simulink model "Safety_filter_taskspace_run_FxTISMC"  (R2022a)
settings: Solver=ode4  StartTime=0.0  StopTime=30  FixedStep=0.01  RelTol=1e-3
libraries: simulink x1
settings Model: PacingRate=0.500000  Creator=14244039  LastModifiedBy=40335991
settings DebuggingCC: UnconnectedInputMsg=warning  UnconnectedOutputMsg=warning  UnconnectedLineMsg=warning  UnderSpecifiedDimensionMsg=warning
settings RTWCC: DLArmComputeVersion=19.05

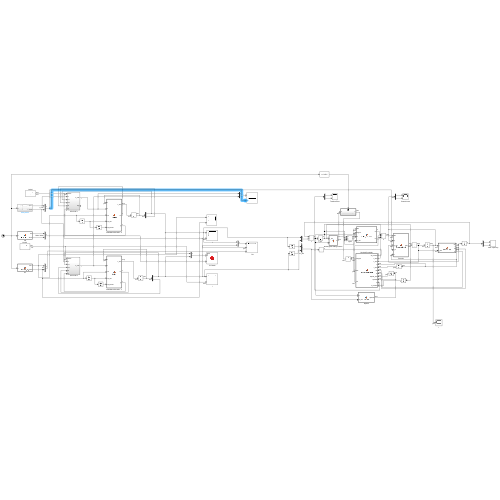
[thumbnail: Simulink's stored preview of the top-level diagram]
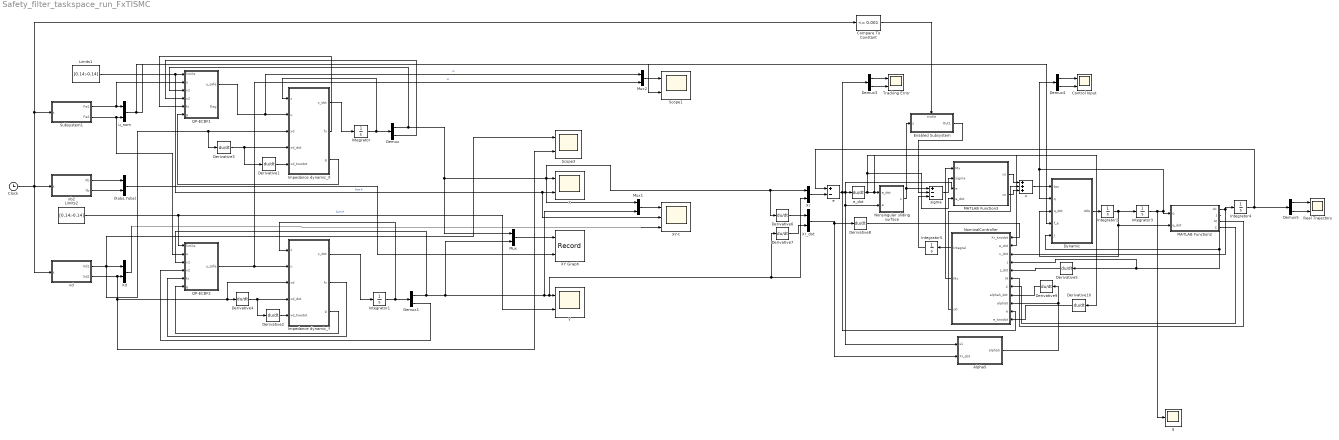
== system Safety_filter_taskspace_run_FxTISMC ==
  " Tracking Error" : Scope  NumInputPorts=2
  (Xobs,Yobs) : Mux  Inputs=2
  AlphaS : MATLAB Function  TreatAsAtomicUnit=on
  Clock : Clock
  Compare To Constant : simulink/Logic and Bit Operations/Compare To Constant  relop=<=  const=0.001  OutDataTypeStr=boolean
  Control Input : Scope  NumInputPorts=2
  Demux{,1,3..5} (5 alike) : Demux  Outputs=2
  Derivative{1..10} (10 alike) : Derivative
  Dynamic : MATLAB Function  TreatAsAtomicUnit=on
  Enabled Subsystem : Subsystem  TreatAsAtomicUnit=on
  Impedance dynamic_X : MATLAB Function  TreatAsAtomicUnit=on
  Impedance dynamic_Y : MATLAB Function  TreatAsAtomicUnit=on
  Integrator : Integrator  InitialCondition=[0.109;0]
  Integrator1 : Integrator  InitialCondition=[0;0]
  Integrator2 : Integrator
  Integrator3 : Integrator  InitialCondition=[0.5236;2.0944]
  Integrator4 : Integrator  InitialCondition=[0.14;0]
  Integrator5 : Integrator  InitialCondition=[0.0001;0.0001]
  Limits1 : Constant  Value=[0.14;-0.14]  VectorParams1D=off  SampleTime=-1
  Limits2 : Constant  Value=[0.14;-0.14]  VectorParams1D=off  SampleTime=-1
  MATLAB Function2 : MATLAB Function  TreatAsAtomicUnit=on
  MATLAB Function3 : MATLAB Function  TreatAsAtomicUnit=on
  Mux : Mux  Inputs=2
  Mux1 : Mux  Inputs=2
  Mux2 : Mux  Inputs=2
  NominalController : MATLAB Function  TreatAsAtomicUnit=on
  Nonsingular sliding surface : MATLAB Function  TreatAsAtomicUnit=on
  QP-ECBF1 : Subsystem
  QP-ECBF2 : Subsystem
  Real Trajectory : Scope  NumInputPorts=2
  Scope1 : Scope  NumInputPorts=2
  Scope3 : Scope  NumInputPorts=2
  Subsystem1 : Subsystem
  X : Scope  NumInputPorts=2
  XY Graph : Record  VariableName=Traj  RecordToWorkspace=on  FileSettingsInternal="{\"entries\":[{\"content\":{\"excelSettings\":{\"content\":{},\"type\":\"Streamout.ExcelSettings\"}},\"type\":\"Streamout.FileSettingStorage\",\"uuid\":\"dea1f68e-51ea-4f94-ad75-dcaf29079ec1\"}],\"packageUris\":[\"http://schema.mathworks.com/mf0/streamout_blocks/R2020a\"],\"version\":\"1.0\"}"  Layout=[1 1]  SignalsInternal="{\"entries\":[{\"content\":{\"signals\":[{\"content\":{\"blockPath\":[\"Safety_filter_taskspace_run_FxTISMC/XY Graph\"],\"channel\":[],\"dimensions\":[2],\"domain\":\"Safety_filter_taskspace_run_FxTISMC/XY Graph\",\"hasChildren\":true,\"lineColor\":\"#0072bd\",\"plots\":[],\"port\":1,\"sid\":[\"\"],\"signalID\":23698,\"signalName\":\"Mux\"},\"type\":\"RecordBlkView.Signal\",\"uuid\":\"0a4beed2-2c3d-4c2f-aacd-e662c2a4948f\"},{\"content\":{\"blockPath\":[\"Safety_filter_taskspace_run_FxTISMC/XY Graph\"],\"channel\":[1],\"dimensions\":[2],\"domain\":\"Safety_filter_taskspace_run_FxTISMC/XY Graph\",\"lineColor\":\"#4dbeee\",\"parentID\":23698,\"plots\":[1],\"port\":1,\"sid\":[\"\"],\"signalID\":23699,\"signalName\":\"Mux\"},\"type\":\"RecordBlkView.Signal\",\"uuid\":\"3713fb18-b151-4fd8-8a41-96ba99eca4e4\"},{\"content\":{\"blockPath\":[\"Safety_filter_taskspace_run_FxTISMC/XY Graph\"],\"channel\":[],\"dimensions\":[2],\"domain\":\"Safety_filter_taskspace_run_FxTISMC/XY Graph\",\"hasChildren\":true,\"lineColor\":\"#edb120\",\"plots\":[],\"port\":2,\"sid\":[\"\"],\"signalID\":23703,\"signalName\":\"(Xobs,Yobs)\"},\"type\":\"RecordBlkView.Signal\",\"uuid\":\"6070feb2-4c26-4461-aa6d-6878fe9a321b\"},{\"content\":{\"blockPath\":[\"Safety_filter_taskspace_run_FxTISMC/XY Graph\"],\"channel\":[1],\"dimensions\":[2],\"domain\":\"Safety_filter_taskspace_run_FxTISMC/XY Graph\",\"lineColor\":\"#139fff\",\"parentID\":23703,\"plots\":[],\"port\":2,\"sid\":[\"\"],\"signalID\":23704,\"signalName\":\"(Xobs,Yobs)\"},\"type\":\"RecordBlkView.Signal\",\"uuid\":\"40400d7a-2fa8-4b38-a7ba-519d3c7263bf\"},{\"content\":{\"blockPath\":[\"Safety_filter_taskspace_run_FxTISMC/XY Graph\"],\"channel\":[2],\"dimensions\":[2],\"domain\":\"Safety_filter_taskspace_run_FxTISMC/XY Graph\",\"lineColor\":\"#ff6929\",\"parentID\":23698,\"plots\":[1],\"port\":1,\"sid\":[\"\"],\"signalID\":23709,\"signalName\":\"Mux\"},\"type\":\"RecordBlkView.Signal\",\"uuid\":\"780f58a9-210e-4d63-889b-484a7d57ccdb\"},{\"content\":{\"blockPath\":[\"Safety_filter_taskspace_run_FxTISMC/XY Graph\"],\"channel\":[2],\"dimensions\":[2],\"domain\":\"Safety_filter_taskspace_run_FxTISMC/XY Graph\",\"lineColor\":\"#b746ff\",\"parentID\":23703,\"plots\":[],\"port\":2,\"sid\":[\"\"],\"signalID\":23710,\"signalName\":\"(Xobs,Yobs)\"},\"type\":\"RecordBlkView.Signal\",\"uuid\":\"fbf2c2ca-e6c1-4b56-8b91-8f9b3b0d1395\"}]},\"type\":\"RecordBlkView.InputSignals\",\"uuid\":\"3059aa5f-a949-4de9-9f01-a09f95338b02\"}],\"packageUris\":[\"http://schema.mathworks.com/mf0/streamout_blocks/R2020a\"],\"version\":\"1.0\"}"  VisualizationBindings="{\"xyplotplugin\":{\"info\":[{\"series\":[{\"bindingParametersList\":[{\"parameter\":\"X-Axis\",\"signalID\":23699,\"signalName\":\"Mux(1)\"},{\"parameter\":\"Y-Axis\",\"signalID\":23709,\"signalName\":\"Mux(2)\"}],\"seriesID\":34366}],\"subplotID\":1}]}}"  CompatibilityTag=XY  st=-1
  XY-t : Scope  NumInputPorts=3
  Xd : Mux  Inputs=2
  Xr : Mux  Inputs=2
  Xr_dot : Mux  Inputs=2
  Y : Scope  NumInputPorts=2
  e : Sum  Inputs=+-
  e_dot : Derivative
  q : Scope
  sigma : Sum  Inputs=+--
  u : Sum  Inputs=+++
  u_nom : Mux  Inputs=2
  xb2 : MATLAB Function  TreatAsAtomicUnit=on
  xd : MATLAB Function  TreatAsAtomicUnit=on
  wires:
  xd/1(Xd1) -> Scope3/1, Impedance dynamic_X/3(xd), Derivative3/1, Xd/1
  Subsystem1/1(Fe1) -> QP-ECBF1/2(u), u_nom/1
  Clock/1 -> xd/1(t), xb2/1(t), Compare To Constant/1, Subsystem1/1(t)
  Derivative3/1 -> Impedance dynamic_X/4(xd_dot), Derivative1/1
  Derivative1/1 -> Impedance dynamic_X/5(xd_twodot)
  Impedance dynamic_X/1(x_dot) -> Integrator/1
  Integrator/1 -> Demux/1, Impedance dynamic_X/1(x)
  Demux/1 -> QP-ECBF1/3(x1), Mux/1, Mux1/1, X/1, Derivative6/1, Xr/1
  Limits1/1 -> XY-t/2, X/2, QP-ECBF1/1(limits)  "lim+"
  Demux/2 -> QP-ECBF1/4(x2)
  QP-ECBF1/1(u_safe) -> Mux2/1, Impedance dynamic_X/2(u)  "u"
  Impedance dynamic_X/2(fx) -> QP-ECBF1/5(fx)
  Impedance dynamic_X/3(g) -> QP-ECBF1/6(g)
  Impedance dynamic_Y/3(g) -> QP-ECBF2/6(g)
  Impedance dynamic_Y/2(fx) -> QP-ECBF2/5(fx)
  QP-ECBF2/1(u_safe) -> Mux2/2, Impedance dynamic_Y/2(u)  "u"
  Demux1/2 -> QP-ECBF2/4(x2)
  Demux1/1 -> QP-ECBF2/3(x1), Mux1/2, Derivative7/1, Xr/2, Y/1, Mux/2
  xd/2(Xd2) -> Scope3/2, Impedance dynamic_Y/3(xd), Derivative4/1, Xd/2
  Limits2/1 -> Y/2, QP-ECBF2/1(limits)  "lim+"
  Impedance dynamic_Y/1(x_dot) -> Integrator1/1
  Derivative4/1 -> Impedance dynamic_Y/4(xd_dot), Derivative2/1
  Derivative2/1 -> Impedance dynamic_Y/5(xd_twodot)
  Integrator1/1 -> Demux1/1, Impedance dynamic_Y/1(x)
  Subsystem1/2(Fe2) -> QP-ECBF2/2(u), u_nom/2
  xb2/1(Xb) -> (Xobs,Yobs)/1
  xb2/2(Yb) -> (Xobs,Yobs)/2
  Mux/1 -> XY Graph/1
  (Xobs,Yobs)/1 -> XY Graph/2
  Mux1/1 -> XY-t/1
  Xd/1 -> XY-t/3
  Mux2/1 -> Scope1/1
  u_nom/1 -> Dynamic/4(f_e), Scope1/2
  Xr/1 -> e/2
  Demux4/2 -> Control Input/2
  Nonsingular sliding surface/1(s) -> Enabled Subsystem/1(s), sigma/1
  Demux3/1 -> " Tracking Error"/1
  Integrator5/1 -> sigma/3
  NominalController/1(Integral) -> Integrator5/1
  Demux5/2 -> Real Trajectory/2
  Compare To Constant/1 -> Enabled Subsystem/Enable
  Demux3/2 -> " Tracking Error"/2
  Derivative7/1 -> Xr_dot/2
  e_dot/1 -> MATLAB Function3/4(e_dot), Derivative10/1, NominalController/2(e_dot), Nonsingular sliding surface/1(e_dot)
  MATLAB Function3/1(us) -> u/1
  Derivative5/1 -> NominalController/5(J_dot)
  Integrator2/1 -> MATLAB Function2/2(q_dot), Dynamic/3(q_dot), Integrator3/1
  Demux5/1 -> Real Trajectory/1
  MATLAB Function2/2(J) -> Dynamic/5(J), NominalController/4(J), Derivative5/1
  Integrator3/1 -> q/1, Demux4/1, Dynamic/2(q), MATLAB Function2/1(q)
  sigma/1 -> MATLAB Function3/2(sigma)
  Integrator4/1 -> Demux5/1, e/1
  Enabled Subsystem/1(Out1) -> sigma/2
  Derivative10/1 -> NominalController/11(e_twodot)
  MATLAB Function2/4(C) -> NominalController/7(C)
  NominalController/3(u0) -> u/2
  Xr_dot/1 -> AlphaS/2(Xr_dot), Derivative8/1
  Derivative9/1 -> NominalController/8(alphaS_dot)
  AlphaS/1(alphaS) -> Derivative9/1, NominalController/9(alphaS)
  MATLAB Function2/3(M) -> NominalController/6(M)
  MATLAB Function3/2(uc) -> u/3
  Derivative6/1 -> Xr_dot/1
  Dynamic/1(ddq) -> Integrator2/1
  NominalController/2(Mx) -> MATLAB Function3/1(Mx)
  Derivative8/1 -> NominalController/1(Xr_twodot)
  e/1 -> Demux3/1, e_dot/1, MATLAB Function3/3(e), AlphaS/1(s1), Nonsingular sliding surface/2(e), NominalController/10(e)
  MATLAB Function2/1(dx) -> Integrator4/1, NominalController/3(x_dot)
  u/1 -> Dynamic/1(tau)
  Demux4/1 -> Control Input/1

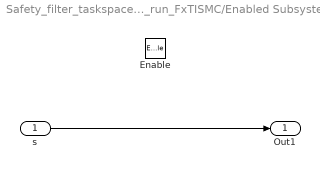
== system Safety_filter_taskspace_run_FxTISMC/Enabled Subsystem ==
  s : Inport
  Enable : EnablePort
  Out1 : Outport  InitialOutput=0  VectorParamsAs1DForOutWhenUnconnected=off
  wires:
  s/1 -> Out1/1

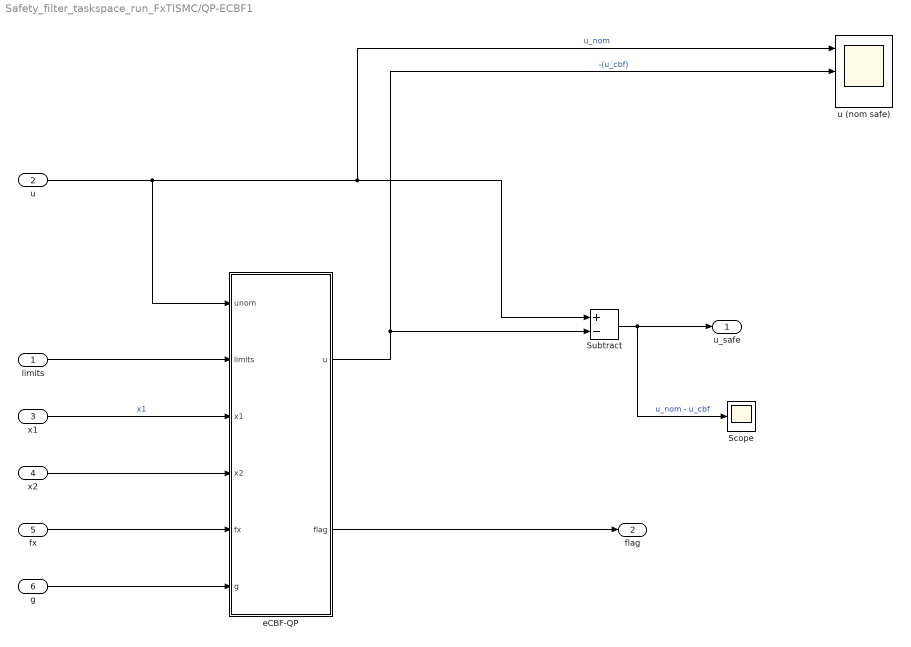
== system Safety_filter_taskspace_run_FxTISMC/QP-ECBF1 ==
  limits : Inport
  u : Inport  Port=2
  x1 : Inport  Port=3
  x2 : Inport  Port=4
  fx : Inport  Port=5
  g : Inport  Port=6
  Scope : Scope
  Subtract : Sum  Inputs=+-
  eCBF-QP : MATLAB Function  TreatAsAtomicUnit=on
  u (nom safe) : Scope  NumInputPorts=3
  u_safe : Outport
  flag : Outport  Port=2
  wires:
  x2/1 -> eCBF-QP/4(x2)
  limits/1 -> eCBF-QP/2(limits)
  u/1 -> eCBF-QP/1(unom), Subtract/1, u (nom safe)/1  "u_nom"
  x1/1 -> eCBF-QP/3(x1)  "x1"
  eCBF-QP/1(u) -> Subtract/2, u (nom safe)/2  "-(u_cbf)"
  Subtract/1 -> u_safe/1, Scope/1  "u_nom - u_cbf"
  fx/1 -> eCBF-QP/5(fx)
  g/1 -> eCBF-QP/6(g)
  eCBF-QP/2(flag) -> flag/1

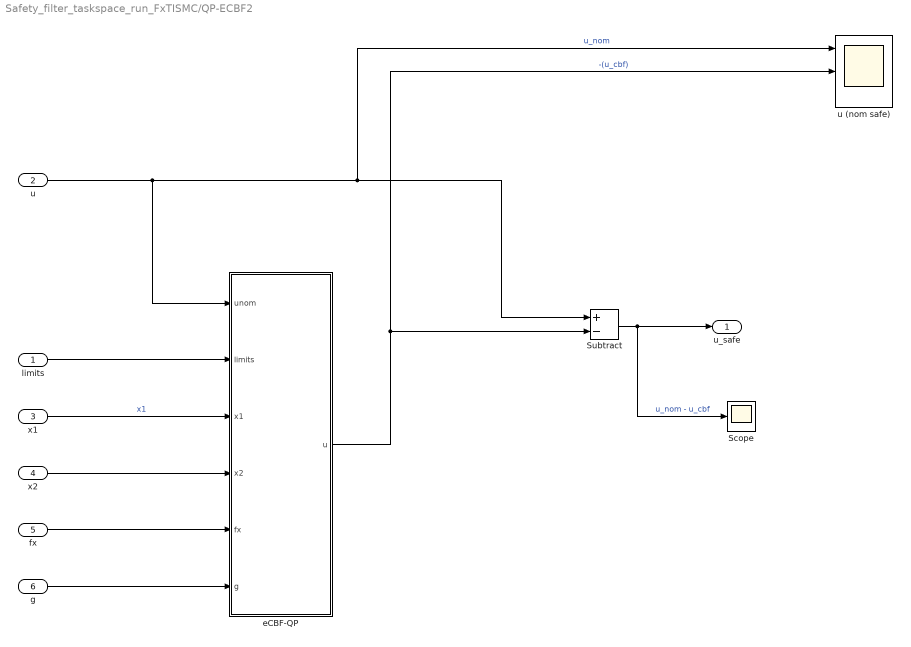
== system Safety_filter_taskspace_run_FxTISMC/QP-ECBF2 ==
  limits : Inport
  u : Inport  Port=2
  x1 : Inport  Port=3
  x2 : Inport  Port=4
  fx : Inport  Port=5
  g : Inport  Port=6
  Scope : Scope
  Subtract : Sum  Inputs=+-
  eCBF-QP : MATLAB Function  TreatAsAtomicUnit=on
  u (nom safe) : Scope  NumInputPorts=3
  u_safe : Outport
  wires:
  x2/1 -> eCBF-QP/4(x2)
  limits/1 -> eCBF-QP/2(limits)
  u/1 -> eCBF-QP/1(unom), Subtract/1, u (nom safe)/1  "u_nom"
  x1/1 -> eCBF-QP/3(x1)  "x1"
  eCBF-QP/1(u) -> Subtract/2, u (nom safe)/2  "-(u_cbf)"
  Subtract/1 -> u_safe/1, Scope/1  "u_nom - u_cbf"
  fx/1 -> eCBF-QP/5(fx)
  g/1 -> eCBF-QP/6(g)

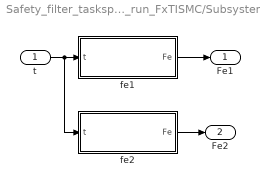
== system Safety_filter_taskspace_run_FxTISMC/Subsystem1 ==
  t : Inport
  fe1 : MATLAB Function  TreatAsAtomicUnit=on
  fe2 : MATLAB Function  TreatAsAtomicUnit=on
  Fe1 : Outport
  Fe2 : Outport  Port=2
  wires:
  fe1/1(Fe) -> Fe1/1
  fe2/1(Fe) -> Fe2/1
  t/1 -> fe2/1(t), fe1/1(t)

== matlab function Safety_filter_taskspace_run_FxTISMC/Dynamic ==
  data: tau input size=[2 1]; ddq output size=[2 1]; q input size=[2 1]; q_dot input size=[2 1]; f_e input; J input
function ddq  = TwoLinkRobot(tau,q,q_dot,f_e,J)
L = [0.3, 0.3];
m = [1.5, 1];
g = 9.8;

M = [m(2)*L(2)^2+2*m(2)*L(1)*L(2)*cos(q(2))+(m(1)+m(2))*L(1)^2, m(2)*L(2)^2+m(2)*L(1)*L(2)*cos(q(2));
    m(2)*L(2)^2+m(2)*L(1)*L(2)*cos(q(2)), m(2)*L(2)^2];
C = [-2*m(2)*L(1)*L(2)*sin(q(2))*q_dot(2), -m(2)*L(1)*L(2)*sin(q(2)); 
    m(2)*L(1)*L(2)*sin(q(2))*q_dot(1), 0];

F=[2*cos(q(1))*sin(q(2))+5*cos(q(1))^2;-2*cos(q(1))*sin(q(2))-5*cos(q(1))^2];

tau_e = (J')*f_e;
ddq = M\(-C*q_dot-F + tau + tau_e);

end

== matlab function Safety_filter_taskspace_run_FxTISMC/AlphaS ==
  data: s1 input; alphaS output; Xr_dot input
function alphaS = AlphaS(s1,Xr_dot)

k1=3;
k2=20;
k3=50;

alpha=5/7;
beta=5/3;

alphaS = -(k1.*s1 + k2.*abs(s1).^alpha.*sign(s1) + k3.*abs(s1).^beta.*sign(s1)) + Xr_dot;

end

== matlab function Safety_filter_taskspace_run_FxTISMC/MATLAB Function2 ==
  data: q input; q_dot input; dx output; J output; M output; C output
function [dx,J,M,C]  = JointTwoTask(q,q_dot)
L = [0.3, 0.3];
m = [1.5, 1];

M = [m(2)*L(2)^2+2*m(2)*L(1)*L(2)*cos(q(2))+(m(1)+m(2))*L(1)^2, m(2)*L(2)^2+m(2)*L(1)*L(2)*cos(q(2));
    m(2)*L(2)^2+m(2)*L(1)*L(2)*cos(q(2)), m(2)*L(2)^2];
C = [-2*m(2)*L(1)*L(2)*sin(q(2))*q_dot(2), -m(2)*L(1)*L(2)*sin(q(2)); 
    m(2)*L(1)*L(2)*sin(q(2))*q_dot(1), 0];
J = [-L(1)*sin(q(1))-L(2)*sin(q(1)+q(2)), -L(2)*sin(q(1)+q(2));
    L(1)*cos(q(1))+L(2)*cos(q(1)+q(2)), L(2)*cos(q(1)+q(2))];
dx = J*q_dot;
end

== matlab function Safety_filter_taskspace_run_FxTISMC/MATLAB Function3 ==
  data: Mx input; us output; sigma input; uc output; e input; e_dot input
function [us,uc] = ISMC_Controller(Mx,sigma,e,e_dot)

K_gain=0.001;
k1=20;
k2=50;
alpha=5/3;
beta=5/7;
Mxx=pinv(Mx);
gamma = 5/7;
us = -inv(Mx)*((K_gain+0.001)*sign(sigma) + k1*abs(sigma).^alpha.*sign(sigma) + k2*abs(sigma).^beta.*sign(sigma));
% uc = -Mxx*k2^gamma*(abs(e_dot+k1*abs(e).^alpha.*sign(e)).^(1/gamma-1)).*e_dot;
uc = 0;
end

== matlab function Safety_filter_taskspace_run_FxTISMC/NominalController ==
  data: Xr_twodot input; e_dot input; x_dot input size=[2 1]; J input; J_dot input; M input; C input; alphaS_dot input size=[2 1]; Integral output size=[2 1]; Mx output size=[2 2]; u0 output size=[2 1]; alphaS input; e input; e_twodot input
function [Integral,Mx,u0] = NominalController(Xr_twodot,e_dot,x_dot,J,J_dot,M,C,alphaS_dot,alphaS,e,e_twodot)

Mx = inv(J')*M*inv(J);
Cx = inv(J')*(C-(M*inv(J)*J_dot))*inv(J);

%% PD Controller
% Kp=35;
% Kd=400;
% f=Mx*(Kp*(Xr-x)+Kd*(Xr_dot-x_dot)) + Cx*x_dot;
% u0=(J')*f;

%% Fixed-time backstepping control
k8=3;
k9=20;
k10=50;
alpha=5/3;
beta=5/7;
gamma = 5/7;

s2 = x_dot - alphaS;

f0 = Mx*(inv(Mx)*Cx*x_dot + alphaS_dot - k8*s2 - k9*abs(s2).^alpha.*sign(s2) - k10*abs(s2).^beta.*sign(s2));
u0=(J')*f0;

%% Integral term of fixed-time integral sliding mode controller

k1=20;
k2=50;
%  Integral = Mx\u0 +  Mx\Cx*x_dot - Xr_twodot + e_dot + (1/k2^gamma)*(abs(e_dot+k1*abs(e).^alpha.*sign(e)).^(1/gamma-1)).*(Mx\u0 +  Mx\Cx*x_dot - Xr_twodot + k1*abs(e).^(alpha-1).*e_dot);
Integral = e_dot + (1/k2^gamma)*(abs(e_dot+k1*abs(e).^alpha.*sign(e)).^(1/gamma-1)).*(Mx\u0 +  Mx\Cx*x_dot - Xr_twodot + k1*abs(e).^(alpha-1).*e_dot);


end

== matlab function Safety_filter_taskspace_run_FxTISMC/xb2 ==
  data: t input; Xb output; Yb output
function [Xb,Yb]  = Obstacles_traj(t)

Xb =  -0.07+0.05*cos(t);
Yb =  -0.05+0.05*sin(t);
    
end

== matlab function Safety_filter_taskspace_run_FxTISMC/Nonsingular sliding surface ==
  data: e_dot input; e input; s output
function s = S(e_dot,e)

k1=20;
k2=50;
alpha=5/3;
beta=5/7;
gamma = 5/7;

s = e + (1/k2^(gamma)).*abs(e_dot+k1*abs(e).^alpha.*sign(e)).^(1/gamma).*sign(e_dot+k1*abs(e).^alpha.*sign(e));

end

== matlab function Safety_filter_taskspace_run_FxTISMC/Impedance dynamic_Y ==
  data: x input size=[2 1]; u input; x_dot output size=[2 1]; xd input; xd_dot input; xd_twodot input; fx output; g output
function [x_dot,fx,g] = System(x,u,xd,xd_dot,xd_twodot)

    km = 20;
    kb = 20;                                                       
    kk = 100;
    fx = [x(2);
        -(1/km)*(kb*(x(2)-xd_dot)+kk*(x(1)-xd)-km*xd_twodot)];
    g = [0;km^(-1)];
    x_dot = fx + g*u;
end

== matlab function Safety_filter_taskspace_run_FxTISMC/Subsystem1/fe1 ==
  data: t input; Fe output
function Fe  = External_force(t)

    Fe = 0*(t<4|t>=11) + (1-cos(pi*t))*(t>=4&t<5) + 2*(t>=5&t<10) + (1+cos(pi*t))*(t>=10&t<11);

end

== matlab function Safety_filter_taskspace_run_FxTISMC/QP-ECBF2/eCBF-QP ==
  settings: updateMethod=DISCRETE
  data: unom input; limits input; u output size=1; x1 input; x2 input; fx input; g input
function u = fcn(unom, limits, x1, x2,fx,g)
 %Barrier Limits
    lim     = limits(1);
    lim2    = limits(2);
 
    %ECBF Gains
    k1      = 50;
    k2      = 300;
    
    k3      = k1;
    k4      = k2;
    % Maximum Value CBF variables
    hx      = (x1 - lim)^2 - 0.001 ;  %(lim^2 - x1^2) 
    Lfhx    = 2*(x1 - lim)*x2;
    
%     L2fhx   = 2*(x1 - lim)*((2*x1*(x1^2 + x2)) + x1*x2 + x1 + (1 + x1^2)*CTL) + 2*(x1^2 + x2)^2;
%     eCBF    = L2fhx + k1*Lfhx + k2*hx;
    
    % Minimum Value CBF variables
    hx2     = (lim2 - x1)^2 - 0.001 ;  %(lim^2 - x1^2) 
    Lfhx2    = -2*(lim2 - x1)*x2;


    H       = [2 0; 0 0];
    f       = [0;0]; 
    
    A       = [2*(x1-lim)*g(2) 0;
              -2*(lim2 - x1)*g(2) 0]; 
            
    b       = [ 2*(x1 - lim) * (  g(2)*unom) + k1*Lfhx + k2*hx;
               -2*(lim2 - x1) * ( g(2)*unom) + k3*Lfhx2 + k4*hx2];
    X   = [0;0];
    flag = 0;
    coder.extrinsic('quadprog');
    [output, ~, flag]   = quadprog(H,f,A,b,[],[],[],[]);

    if flag == 1
        X = output;
    else
        X   = [0;0];
    end
    
%Function outputs
    u = X(1); 
end

== matlab function Safety_filter_taskspace_run_FxTISMC/Subsystem1/fe2 ==
  data: t input; Fe output
function Fe  = External_force(t)

   Fe = 0*(t<4|t>=11) + 2*(1-cos(pi*t))*(t>=4&t<5) + 4*(t>=5&t<10) + 2*(1+cos(pi*t))*(t>=10&t<11);

end

== matlab function Safety_filter_taskspace_run_FxTISMC/xd ==
  data: t input; Xd1 output; Xd2 output
function [Xd1, Xd2] = Desired_traj(t)

    Xd1=0.14*cos(0.5*t);
    Xd2=0.14*sin(0.5*t);
    
end

== matlab function Safety_filter_taskspace_run_FxTISMC/QP-ECBF1/eCBF-QP ==
  settings: updateMethod=DISCRETE
  data: unom input; limits input; u output size=1; x1 input; x2 input; fx input; g input; flag output
function [u,flag] = fcn(unom, limits, x1, x2,fx,g)
     %Barrier Limits
    lim     = limits(1);
    lim2    = limits(2);
 
    %ECBF Gains
    k1      = 50;
    k2      = 300;
    
    k3      = k1;
    k4      = k2;
    % Maximum Value CBF variables
    hx      = (x1 - lim)^2 - 0.001 ;  %(lim^2 - x1^2) 
    Lfhx    = 2*(x1 - lim)*x2;
    
%     L2fhx   = 2*(x1 - lim)*((2*x1*(x1^2 + x2)) + x1*x2 + x1 + (1 + x1^2)*CTL) + 2*(x1^2 + x2)^2;
%     eCBF    = L2fhx + k1*Lfhx + k2*hx;
    
    % Minimum Value CBF variables
    hx2     = (lim2 - x1)^2 - 0.001 ;  %(lim^2 - x1^2) 
    Lfhx2    = -2*(lim2 - x1)*x2;


    H       = [2 0; 0 0];
    f       = [0;0]; 
    
    A       = [2*(x1-lim)*g(2) 0;
              -2*(lim2 - x1)*g(2) 0]; 
            
    b       = [ 2*(x1 - lim) * ( g(2)*unom) + k1*Lfhx + k2*hx;
               -2*(lim2 - x1) * (  g(2)*unom)  + k3*Lfhx2 + k4*hx2];
    X   = [0;0];
    flag = 0;
    coder.extrinsic('quadprog');
    [output, ~, flag]   = quadprog(H,f,A,b,[],[],[],[]);

    if flag == 1
        X = output;
    else
        X   = [0;0];
    end
    
%Function outputs
    u = X(1); 
end

== matlab function Safety_filter_taskspace_run_FxTISMC/Impedance dynamic_X ==
  data: x input size=[2 1]; u input; x_dot output size=[2 1]; xd input; xd_dot input; xd_twodot input; fx output; g output
function [x_dot,fx,g] = System(x,u,xd,xd_dot,xd_twodot)

    km = 20;
    kb = 20;                                                       
    kk = 100;
    fx = [x(2);
        -(1/km)*(kb*(x(2)-xd_dot)+kk*(x(1)-xd)-km*xd_twodot)];
    g = [0;km^(-1)];
    x_dot = fx + g*u;
end
